simulink model "ExampleDriveInternalPhysics"  (R2024b)
settings: Solver=FixedStepDiscrete  StartTime=0.0  StopTime=inf  FixedStep=0.001  RelTol=1e-3  EnableMultiTasking=on
libraries: rFproPhysicsLib x3
settings Model: Creator=enewton  LastModifiedBy=Saian
settings SolverCC: AlgebraicLoopSolver=TrustRegion
settings DataIOCC: LimitDataPoints=on  SaveFormat=Array  SignalLoggingSaveFormat=ModelDataLogs  ReturnWorkspaceOutputs=off
settings OptimizationCC: ExpressionDepthLimit=2147483647  EfficientFloat2IntCast=on  LifeSpan=inf
settings DebuggingCC: UnderspecifiedInitializationDetection=Classic  MergeDetectMultiDrivingBlocksExec=none  SolverPrmCheckMsg=warning  FcnCallInpInsideContextMsg=warning  UnconnectedInputMsg=warning  UnconnectedOutputMsg=warning  UnconnectedLineMsg=warning  StateNameClashWarn=warning  SFUnexpectedBacktrackingDiag=warning  SFNoUnconditionalDefaultTransitionDiag=warning  SFExecutionAtInitializationDiag=none  ArithmeticOperatorsInVariantConditions=warning
settings HardwareCC: ProdBitPerPointer=32  ProdBitPerSizeT=32  ProdBitPerPtrDiffT=32  ProdLargestAtomicFloat=None  ProdIntDivRoundTo=Undefined  ProdEndianess=Unspecified  ProdWordSize=32  ProdHWDeviceType=32-bit Generic
settings ModelReferenceCC: EnableRefExpFcnMdlSchedulingChecks=on  PropagateSignalLabelsOutOfModel=off
settings SFSimCC: SimUseLocalCustomCode=off  CustomCodeUndefinedFunction=UseInterfaceOnly  SimTargetLang=C++
settings RTWCC: Description=rFpro Target (Run Physics)  SystemTargetFile=rfpro.tlc  MakeCommand="make_rtw OPTS=\"-DRUN_PHYSICS\""  TemplateMakefile=rfpro.tmf  RTWUseLocalCustomCode=off  TargetLang=C++  GPUComputeCapability=3.5
settings CodeAppCC: StateflowObjectComments=on
settings STFCustomTargetCC: ModelReferenceCompliant=off  CombineOutputUpdateFcns=on  MatFileLogging=on  CPPClassGenCompliant=on  SystemTargetFile=rfpro.tlc
settings GRTTargetCC: TargetLangStandard=C89/C90 (ANSI)  ModelReferenceCompliant=off  ParMdlRefBuildCompliant=off  CompOptLevelCompliant=off  ConcurrentExecutionCompliant=off  UseToolchainInfoCompliant=off
settings ConfigComp: CovMetricSettings=dw  CovSaveCumulativeToWorkspaceVar=on  CovSaveSingleToWorkspaceVar=on  CovExternalEMLEnable=off

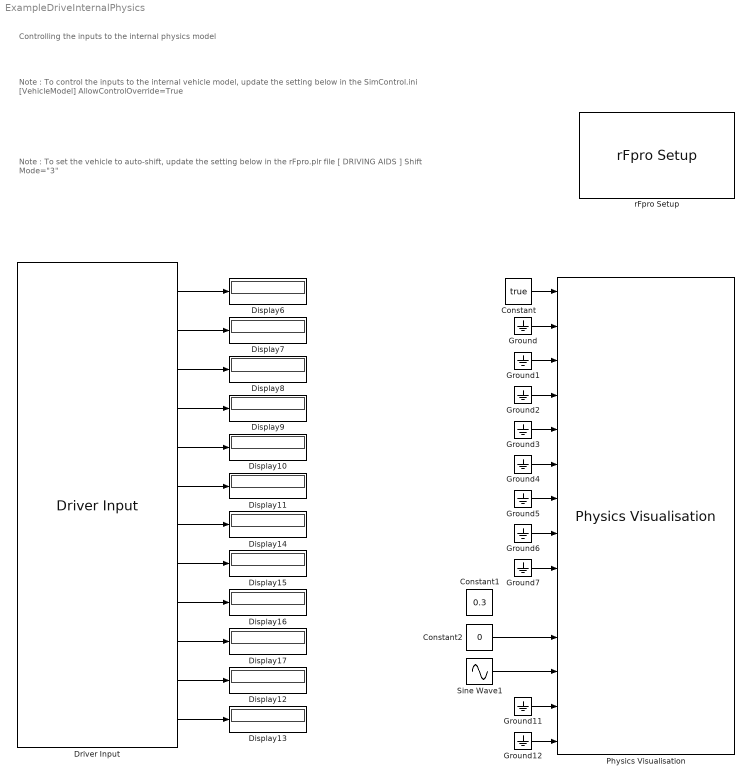
== system ExampleDriveInternalPhysics ==
  note: Note : To set the vehicle to auto-shift, update the setting below in the rFpro.plr file
      |
      | [ DRIVING AIDS ]
      | Shift Mode="3"
  note: Controlling the inputs to the internal physics model
  note: Note : To control the inputs to the internal vehicle model, update the setting below in the SimControl.ini
      |
      | [VehicleModel]
      | AllowControlOverride=True
  Constant : Constant  Value=true
  Constant1 : Constant  Value=0.3
  Constant2 : Constant  Value=0
  Display{6..17} (12 alike) : Display
  Driver Input : rFproPhysicsLib/Driver Input
      settings: SourceProductName=rFpro Physics
  Ground{,1..7,11..12} (10 alike) : Ground
  Physics Visualisation : rFproPhysicsLib/Physics Visualisation  PAR_SKIP_INTERNAL_PHYSICS=off  PAR_ACCEL_VALID=off  PAR_ROT_ACCEL_VALID=off  PAR_GEAR_VALID=off  PAR_RPM_VALID=off  PAR_INPUTS_VALID=on  PAR_STEER_TORQUE_VALID=off  PAR_HEADLIGHTS_ON_VALID=off  PAR_WHEEL_POS_VALID=off  PAR_WHEEL_ORI_VALID=off  PAR_TYRE_PARAMS_VALID=off  PAR_WHEEL_ROTATION_VALID=off  PAR_WHEEL_BRAKE_TEMP_VALID=off  PAR_WHEEL_TREAD_TEMP_VALID=off  PAR_WHEEL_AIR_TEMP_VALID=off  period=-1  offset=0  useReverseByteOrder=on  rFpro__platform=Remote Model - Default
      settings: SourceProductName=rFpro Physics
  Sine Wave1 : Sin  Frequency=0.5  Phase=pi/2  SampleTime=0
  rFpro Setup : rFproPhysicsLib/rFpro Setup  platform=Remote Model - Default  stopOnSessionEnd=on  usePseudoRealtime=on  syncToRF=on  useReverseByteOrder=off  useRfTime=on  minIterations=4  maxIterations=1000  ipReceiveAddress='127.0.0.1'  ipReceivePort=11054  receiveSampleTime=-1  ipTransmitAddress='127.0.0.1'  ipTransmitPort=11052  transmitSampleTime=-1  pluginType=RUN_PHYSICS  sysTarget=xpctarget.tlc  templateMakeFile=xpc_default_tmf  makeCommand=make_rtw  buildDesc=xPC target
      settings: SourceProductName=rFpro Physics
  wires:
  Constant/1 -> Physics Visualisation/1
  Ground/1 -> Physics Visualisation/2
  Ground1/1 -> Physics Visualisation/3
  Ground2/1 -> Physics Visualisation/4
  Ground3/1 -> Physics Visualisation/5
  Ground4/1 -> Physics Visualisation/6
  Ground5/1 -> Physics Visualisation/7
  Ground6/1 -> Physics Visualisation/8
  Ground7/1 -> Physics Visualisation/9
  Constant2/1 -> Physics Visualisation/11
  Sine Wave1/1 -> Physics Visualisation/12
  Ground11/1 -> Physics Visualisation/13
  Ground12/1 -> Physics Visualisation/14
  Driver Input/1 -> Display6/1
  Driver Input/2 -> Display7/1
  Driver Input/3 -> Display8/1
  Driver Input/4 -> Display9/1
  Driver Input/5 -> Display10/1
  Driver Input/6 -> Display11/1
  Driver Input/7 -> Display14/1
  Driver Input/8 -> Display15/1
  Driver Input/9 -> Display16/1
  Driver Input/10 -> Display17/1
  Driver Input/11 -> Display12/1
  Driver Input/12 -> Display13/1
